simulink model "Autopilot_mdl"  (R2018b)
settings: Solver=VariableStepAuto  StartTime=0.0  StopTime=1  MaxStep=0.001  RelTol=1e-3  EnableMultiTasking=on
libraries: lpvlibrary x3, simulink x1
settings Model: Creator=Fernando  LastModifiedBy=ferna
settings OptimizationCC: LifeSpan=inf
settings DebuggingCC: SFUnexpectedBacktrackingDiag=warning  SFNoUnconditionalDefaultTransitionDiag=warning
settings SFSimCC: SimUseLocalCustomCode=off
settings RTWCC: RTWUseLocalCustomCode=off
settings CodeAppCC: StateflowObjectComments=on
settings GRTTargetCC: TargetLangStandard=C89/C90 (ANSI)  GeneratePreprocessorConditionals=Disable all
settings ConfigComp: CovMetricSettings=dw  CovHtmlReporting=on  CovSaveCumulativeToWorkspaceVar=on  CovSaveSingleToWorkspaceVar=on  CovExternalEMLEnable=off

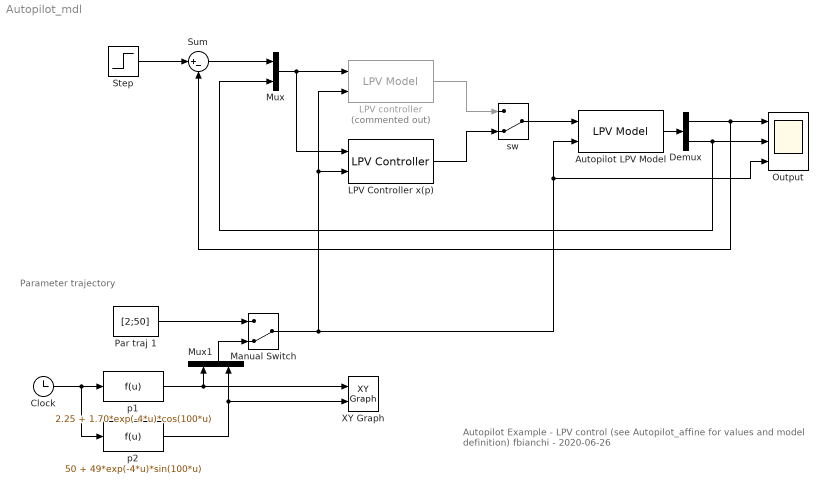
== system Autopilot_mdl ==
  note: Autopilot Example - LPV control
      | (see Autopilot_affine for values and model definition)
      | fbianchi - 2020-06-26
  note: Parameter trajectory
  Autopilot LPV Model : lpvlibrary/LPV Model  pdSys=pdG  x0=0
      settings: SourceProductName=LPV Toolbox
  Clock : Clock
  Demux : Demux  Outputs=2
  LPV Controller x(p) : lpvlibrary/LPV Controller  pdSys=pdK  x0=0
      settings: SourceProductName=LPV Toolbox
  LPV controller : lpvlibrary/LPV Model  Commented=on  pdSys=pdK1  x0=0
      settings: SourceProductName=LPV Toolbox
  Manual Switch : ManualSwitch  CurrentSetting=0
  Mux : Mux  Inputs=2
  Mux1 : Mux  Inputs=2
  Output : Scope  NumInputPorts=3
  Par traj 1 : Constant  Value=[2;50]
  Step : Step  Time=0.2  SampleTime=0
  Sum : Sum  Inputs=|+-
  XY Graph : simulink/Sinks/XY Graph  xmin=0  xmax=5  ymin=0  ymax=110  st=-1
  p1 : Fcn  Expr=2.25 + 1.70*exp(-4*u)*cos(100*u)
  p2 : Fcn  Expr=50 + 49*exp(-4*u)*sin(100*u)
  sw : ManualSwitch  CurrentSetting=0
  wires:
  Autopilot LPV Model/1 -> Demux/1
  Demux/1 -> Sum/2, Output/1
  Demux/2 -> Mux/2, Output/2
  Step/1 -> Sum/1
  Mux/1 -> LPV Controller x(p)/1, LPV controller/1
  Sum/1 -> Mux/1
  Clock/1 -> p2/1, p1/1
  p1/1 -> XY Graph/1, Mux1/1
  p2/1 -> XY Graph/2, Mux1/2
  Mux1/1 -> Manual Switch/2
  Par traj 1/1 -> Manual Switch/1
  Manual Switch/1 -> LPV Controller x(p)/2, LPV controller/2, Output/3, Autopilot LPV Model/2
  sw/1 -> Autopilot LPV Model/1
  LPV controller/1 -> sw/1
  LPV Controller x(p)/1 -> sw/2
